simulink subsystem "testOPT"  (R2020a)
settings: Solver=VariableStepAuto  StartTime=0.0  StopTime=10.0  RelTol=1e-3
libraries: simulink x8
settings Model: Creator=Lamarre  LastModifiedBy=Lamarre

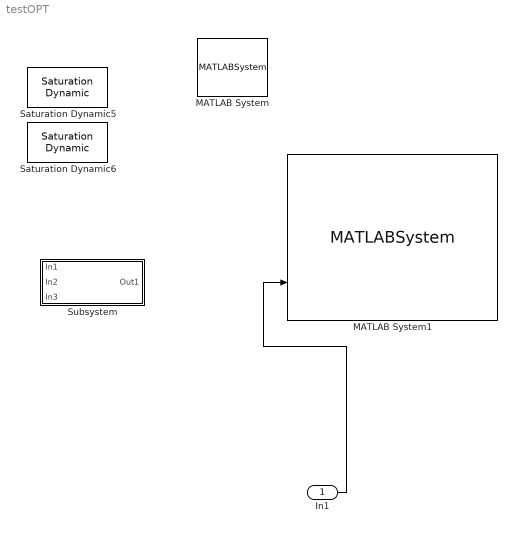
== system testOPT ==
  In1 : Inport
  MATLAB System : MATLABSystem  System=Untitled7  SimulateUsing=Code generation
      mask Type: Untitled7
      mask Display:
      | disp('Untitled7');
      | port_label('input',1,'u');
      | port_label('output',1,'y');
  MATLAB System1 : MATLABSystem  System=Untitled9  L=[]  D=[]  T=[]  FT=[]  MLDT=[]  MLDR=[]  fl=[]  CT=[]  OPT=[]  APX=[]  C=[]  SimulateUsing=Code generation
      mask Type: Untitled9
      mask Display:
      | disp('Untitled9');
      | port_label('input',1,'commande');
      | port_label('input',2,'config');
      | port_label('output',1,'t1');
      | port_label('output',2,'t2');
      | port_label('output',3,'t3');
      | port_label('output',4,'t4');
      | port_label('output',5,'t5');
      | port_label('output',6,'t6');
      | port_label('output',7,'t7');
      | port_label('output',8,'t8');
  Saturation Dynamic5 : simulink/Discontinuities/Saturation Dynamic  OutMin=[]  OutMax=[]  OutDataTypeStr=Inherit: Same as second input  OutDataType=fixdt(1, 16)  OutScaling=2^-10  DoSatur=off
  Saturation Dynamic6 : simulink/Discontinuities/Saturation Dynamic  OutMin=[]  OutMax=[]  OutDataTypeStr=Inherit: Same as second input  OutDataType=fixdt(1, 16)  OutScaling=2^-10  DoSatur=off
  Subsystem : Subsystem
  wires:
  In1/1 -> MATLAB System1/2

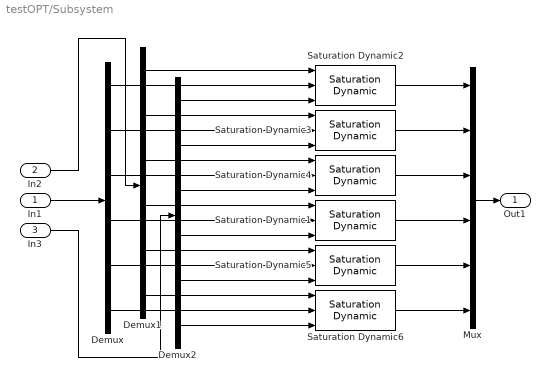
== system testOPT/Subsystem ==
  In1 : Inport
  In2 : Inport  Port=2
  In3 : Inport  Port=3
  Demux : Demux  Outputs=6
  Demux1 : Demux  Outputs=6
  Demux2 : Demux  Outputs=6
  Mux : Mux  Inputs=6
  Saturation Dynamic{1..6} (6 alike) : simulink/Discontinuities/Saturation Dynamic  OutMin=[]  OutMax=[]  OutDataTypeStr=Inherit: Same as second input  OutDataType=fixdt(1, 16)  OutScaling=2^-10  DoSatur=off
  Out1 : Outport
  wires:
  Mux/1 -> Out1/1
  Saturation Dynamic2/1 -> Mux/1
  Saturation Dynamic3/1 -> Mux/2
  Saturation Dynamic4/1 -> Mux/3
  Saturation Dynamic1/1 -> Mux/4
  Demux/1 -> Saturation Dynamic2/2
  Demux/2 -> Saturation Dynamic3/2
  Demux/3 -> Saturation Dynamic4/2
  Demux/4 -> Saturation Dynamic1/2
  Demux/5 -> Saturation Dynamic5/2
  Demux/6 -> Saturation Dynamic6/2
  In1/1 -> Demux/1
  Saturation Dynamic5/1 -> Mux/5
  Saturation Dynamic6/1 -> Mux/6
  Demux1/1 -> Saturation Dynamic2/1
  Demux1/2 -> Saturation Dynamic3/1
  Demux1/3 -> Saturation Dynamic4/1
  Demux1/4 -> Saturation Dynamic1/1
  Demux1/5 -> Saturation Dynamic5/1
  Demux1/6 -> Saturation Dynamic6/1
  In2/1 -> Demux1/1
  In3/1 -> Demux2/1
  Demux2/1 -> Saturation Dynamic2/3
  Demux2/2 -> Saturation Dynamic3/3
  Demux2/3 -> Saturation Dynamic4/3
  Demux2/4 -> Saturation Dynamic1/3
  Demux2/5 -> Saturation Dynamic5/3
  Demux2/6 -> Saturation Dynamic6/3
